simulink library "normalizeBasisParameters"  (R2018a)
settings: Solver=VariableStepAuto  StartTime=0.0  StopTime=10.0  RelTol=1e-3
undefined symbols (not defined in the file): ctrl
settings Model: Creator=M.Cobb  LastModifiedBy=M.Cobb

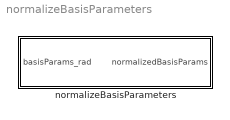
== system normalizeBasisParameters ==
  normalizeBasisParameters : Subsystem

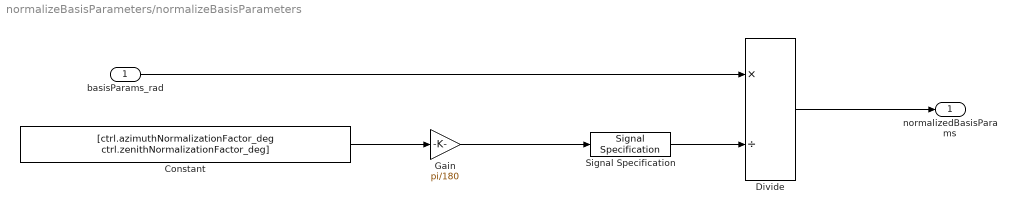
== system normalizeBasisParameters/normalizeBasisParameters ==
  basisParams_rad : Inport  PortDimensions=[1 2]
  Constant : Constant  Value=[ctrl.azimuthNormalizationFactor_deg ctrl.zenithNormalizationFactor_deg]
  Divide : Product  Inputs=*/
  Gain : Gain  Gain=pi/180
  Signal Specification : SignalSpecification  Dimensions=[1 2]
  normalizedBasisParams : Outport  PortDimensions=[1 2]
  wires:
  basisParams_rad/1 -> Divide/1
  Divide/1 -> normalizedBasisParams/1
  Constant/1 -> Gain/1
  Gain/1 -> Signal Specification/1
  Signal Specification/1 -> Divide/2
